simulink model "MotorControl_1"  (Simulink 8.1)
settings: Solver=FixedStepDiscrete  StartTime=0.0  StopTime=100  FixedStep=0.5  RelTol=1e-3
undefined symbols (not defined in the file or in its folder): A14, B, B13, D, L3, R10
libraries: BAMLIB564xL x5, rappid_564xl_ec_toolbox x1
settings Model: Creator=evarshavskaya  LastModifiedBy=evarshavskaya
settings DataIOCC: ExternalInput=off  InitialState=off  SaveOutput=off  SignalLogging=off  SaveTime=off
settings OptimizationCC: InlineParams=on  OptimizeModelRefInitCode=on  LifeSpan=1
settings DebuggingCC: InheritedTsInSrcMsg=none  SingleTaskRateTransMsg=error  UnconnectedInputMsg=error  UnconnectedOutputMsg=error  UnconnectedLineMsg=error  UnknownTsInhSupMsg=error
settings HardwareCC: ProdLargestAtomicInteger=Long  ProdLargestAtomicFloat=Double  ProdIntDivRoundTo=Zero  ProdEndianess=BigEndian  ProdHWDeviceType=Freescale->32-bit PowerPC
settings RTWCC: SystemTargetFile=rappid564xl.tlc  MakeCommand=rappid_564xl_make_rtw  TemplateMakefile=rappid_564xl_default_tmf  PostCodeGenCommand=rappid_analyzegencode(buildInfo)  Description=RAppID Toolbox MPC564xL Code Generation Target (rappid)  ProcessScript=rappid564xl_make_rtw_hook
settings CodeAppCC: IgnoreCustomStorageClasses=off  CustomSymbolStrType=$N$R$M  InternalIdentifier=Classic
settings STFCustomTargetCC: CodeReplacementLibrary=ANSI_C  ModelReferenceCompliant=off  CombineOutputUpdateFcns=on  SuppressErrorStatus=on  ERTCustomFileBanners=on  SupportContinuousTime=off  SupportNonInlinedSFcns=off  MATLABClassNameForMDSCustomization=Simulink.SoftwareTarget.ERTCustomization  GRTInterface=off  SystemTargetFile=rappid564xl.tlc
settings ERTTargetCC: CodeReplacementLibrary=ANSI_C  MultiwordLength=2048  ModelReferenceCompliant=off  ParMdlRefBuildCompliant=off  CompOptLevelCompliant=off  ConcurrentExecutionCompliant=off  SuppressErrorStatus=on  ERTFirstTimeCompliant=off  ModelStepFunctionPrototypeControlCompliant=off  CPPClassGenCompliant=off  ExtModeMexFile=noextcomm  InlinedParameterPlacement=NonHierarchical  ERTCustomFileTemplate=example_file_process.tlc  ConvertIfToSwitch=off  SuppressUnreachableDefaultCases=off

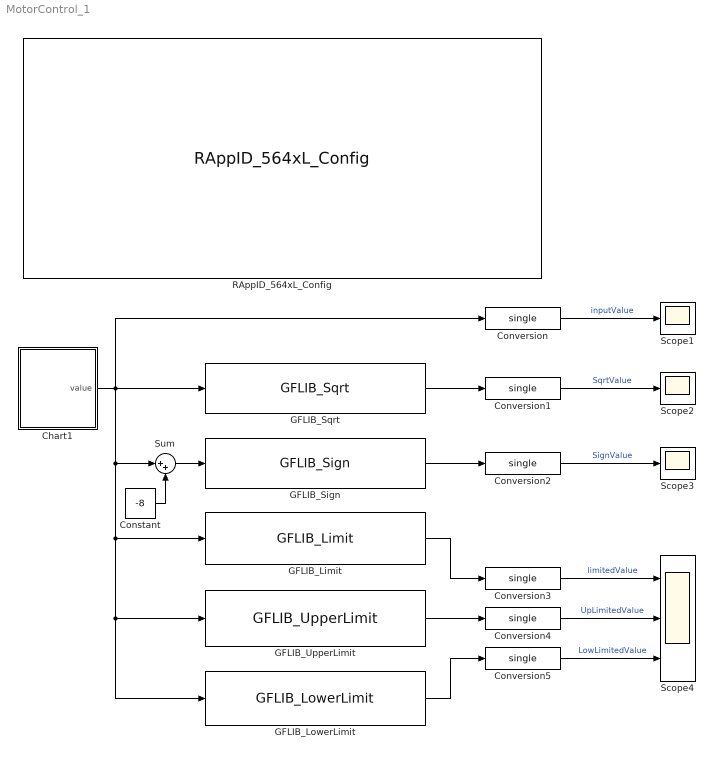
== system MotorControl_1 ==
  Chart1 : Stateflow chart  TreatAsAtomicUnit=on
  Constant : Constant  Value=-8  OutDataTypeStr=single
  Conversion{,1..5} (6 alike) : DataTypeConversion  OutDataTypeStr=single
  GFLIB_Limit : BAMLIB564xL/General Functions/GFLIB_Limit  s32UpperLimit=14  s32LowerLim=2
  GFLIB_LowerLimit : BAMLIB564xL/General Functions/GFLIB_LowerLimit  s32LowerLim=2
  GFLIB_Sign : BAMLIB564xL/General Functions/GFLIB_Sign
  GFLIB_Sqrt : BAMLIB564xL/General Functions/GFLIB_Sqrt
  GFLIB_UpperLimit : BAMLIB564xL/General Functions/GFLIB_UpperLimit  s32UpperLim=14
  RAppID_564xL_Config : rappid_564xl_ec_toolbox/MPC564xL/RAppID_564xL_Config  SystemClock=120  XTAL=40  MC_clock_60=12  MC_clock_80=16  MC_clock_120=10  SWG_clock_60=20  SWG_clock_80=13.334  SWG_clock_120=20  Compiler=CodeWarrior  MemTarget=RAM  Part=MPC5643L  Package=144 LQFP  global_int_priority=10  base_tick_priority=14  sys_task_supress=off  exception_handlers=off  stored_mdl_name=MotorControl_1  freemaster_interface=Oops  freemaster_rx_pin="LINFlex_0 Rx Pin 116 : \"PB[3]\""  freemaster_tx_pin="LINFlex_0 Tx Pin 114 : \"PB[2]\""  freemaster_interface_1=Serial 0  freemaster_enable=on  freemaster_rate=57600  freemaster_tx0_pin=18 : B[2] : 114 : A14  freemaster_rx0_pin=19 : B[3] : 116 : B13  freemaster_tx1_pin=57 : D[9] : 26 : L3  freemaster_rx1_pin=29 : B[13] : 60 : R10  freemaster_can_channel=1CH  freemater_can_speed=500K  freemaster_can_msgig=0x7AA  ccp_interface=None  ccp_enable=off  ccp_can_channel=CH1 (MB 0 - 1)  ccp_can_speed=500K  ccp_can_cro_id=256  ccp_can_dto_id=257  ccp_dev_id=RappID  ccp_dev_addr=0  ccp_odt=3  ccp_daq=3  pil_enable=off  pil_bam=on  comport=1  pil_rate=57600  bam_password_def=on  bam_password=0xFEEDFACECAFEBEEF  bam_sa_cs=off  bam_start_address=0x0  bam_code_size=0x7000  cons_dspi=on  cons_can=on  cons_adc=on  cons_pwm=on  cons_ctu=on  cons_swg=on  cons_eTimer=on  cons_fm=on
  Scope1 : Scope
      settings: TickLabels=on  TimeRange=100  YMin=0  YMax=16
  Scope2 : Scope
      settings: TickLabels=on  TimeRange=100  YMin=0  YMax=4
  Scope3 : Scope
      settings: TickLabels=on  TimeRange=100  YMin=-1  YMax=1  SaveName=ScopeData2
  Scope4 : Scope  NumInputPorts=3
      settings: TickLabels=on  TimeRange=100  YMin=0~0~0  YMax=16~16~16  SaveName=ScopeData3
  Sum : Sum  Inputs=|++
  wires:
  Chart1/1(value) -> GFLIB_Sqrt/1, Sum/1, GFLIB_Limit/1, GFLIB_UpperLimit/1, GFLIB_LowerLimit/1, Conversion/1
  GFLIB_Sqrt/1 -> Conversion1/1
  GFLIB_Sign/1 -> Conversion2/1
  Sum/1 -> GFLIB_Sign/1
  Constant/1 -> Sum/2
  GFLIB_UpperLimit/1 -> Conversion4/1
  GFLIB_Limit/1 -> Conversion3/1
  GFLIB_LowerLimit/1 -> Conversion5/1
  Conversion/1 -> Scope1/1  "inputValue"
  Conversion1/1 -> Scope2/1  "SqrtValue"
  Conversion2/1 -> Scope3/1  "SignValue"
  Conversion4/1 -> Scope4/2  "UpLimitedValue"
  Conversion3/1 -> Scope4/1  "limitedValue"
  Conversion5/1 -> Scope4/3  "LowLimitedValue"

== stateflow chart Chart1 ==
  settings: executeAtInitialization=1
  state A
    du:
    value=cntr;
    cntr=cntr+0.5;
    ex:
    cntr = 0;
  (default) -> A : {cntr=0;}
  A -> A : [cntr >= 16]
  data: cntr local single [0..20] =0; value output single [0..20]
